simulink model "VAB_Linear_Discrete_Piffo"  (R2019b)
settings: Solver=VariableStepAuto  StartTime=0.0  StopTime=t_end  FixedStep=Ts  RelTol=1e-3
undefined symbols (not defined in the file): A_real, B_real, C_real, phi_p_setpoint, Ts, x_0
settings Model: EnablePacing=on  PacingRate=0.045000  Creator=miche  LastModifiedBy=miche

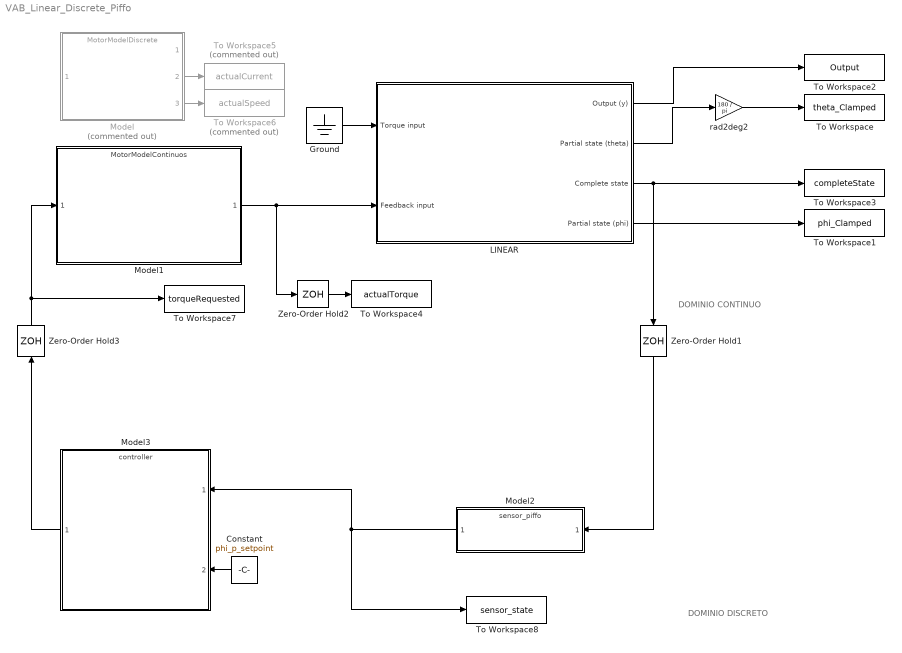
== system VAB_Linear_Discrete_Piffo ==
  note: DOMINIO CONTINUO
  note: DOMINIO DISCRETO
  Constant : Constant  Value=phi_p_setpoint
  Ground : Ground
  LINEAR : Subsystem
  Model : ModelReference  Commented=on  ModelNameDialog=MotorModelDiscrete.slx  SimulationMode=Normal  ModelReferenceVersion=1.14
  Model1 : ModelReference  ModelNameDialog=MotorModelContinuos.slx  SimulationMode=Normal  ModelReferenceVersion=1.24
  Model2 : ModelReference  ModelNameDialog=sensor_piffo.slx  SimulationMode=Normal  ModelReferenceVersion=1.14
  Model3 : ModelReference  ModelNameDialog=controller.slx  SimulationMode=Normal  ModelReferenceVersion=1.20
  To Workspace : ToWorkspace  VariableName=theta_Clamped  SampleTime=-1
  To Workspace1 : ToWorkspace  VariableName=phi_Clamped  SampleTime=-1
  To Workspace2 : ToWorkspace  VariableName=Output  SampleTime=-1
  To Workspace3 : ToWorkspace  VariableName=completeState  SampleTime=-1
  To Workspace4 : ToWorkspace  VariableName=actualTorque  SampleTime=-1
  To Workspace5 : ToWorkspace  Commented=on  VariableName=actualCurrent  SampleTime=-1
  To Workspace6 : ToWorkspace  Commented=on  VariableName=actualSpeed  SampleTime=-1
  To Workspace7 : ToWorkspace  VariableName=torqueRequested  SampleTime=-1
  To Workspace8 : ToWorkspace  VariableName=sensor_state  SampleTime=-1
  Zero-Order Hold1 : ZeroOrderHold  SampleTime=Ts
  Zero-Order Hold2 : ZeroOrderHold  SampleTime=Ts
  Zero-Order Hold3 : ZeroOrderHold  SampleTime=Ts
  rad2deg2 : Gain  Gain=180 / pi
  wires:
  LINEAR/2(Partial state (theta)) -> rad2deg2/1
  LINEAR/1(Output (y)) -> To Workspace2/1
  LINEAR/3("Complete state ") -> Zero-Order Hold1/1, To Workspace3/1
  LINEAR/4(Partial state (phi)) -> To Workspace1/1
  rad2deg2/1 -> To Workspace/1
  Model/2 -> To Workspace5/1
  Model/3 -> To Workspace6/1
  Model3/1 -> Zero-Order Hold3/1
  Model1/1 -> LINEAR/2(Feedback input), Zero-Order Hold2/1
  Zero-Order Hold2/1 -> To Workspace4/1
  Zero-Order Hold1/1 -> Model2/1
  Constant/1 -> Model3/2
  Zero-Order Hold3/1 -> To Workspace7/1, Model1/1
  Ground/1 -> LINEAR/1(Torque input)
  Model2/1 -> To Workspace8/1, Model3/1

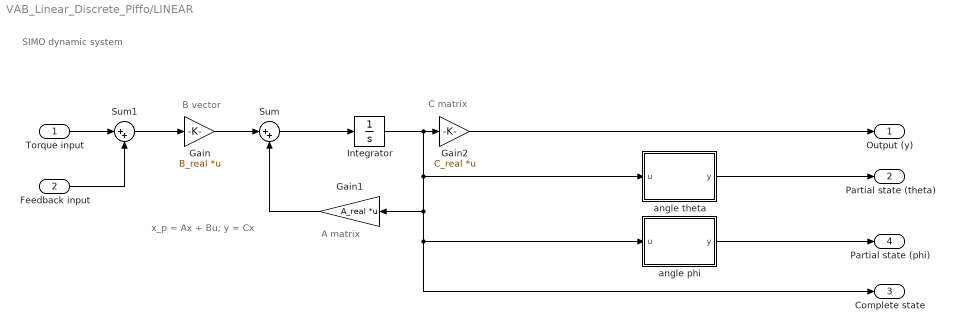
== system VAB_Linear_Discrete_Piffo/LINEAR ==
  note: C matrix
  note: SIMO dynamic system
  note: x_p = Ax + Bu;
      | y = Cx
  note: B vector
  note: A matrix
  Torque input : Inport
  Feedback input : Inport  Port=2
  Gain : Gain  Gain=B_real  Multiplication=Matrix(K*u) (u vector)
  Gain1 : Gain  Gain=A_real  Multiplication=Matrix(K*u) (u vector)
  Gain2 : Gain  Gain=C_real  Multiplication=Matrix(K*u) (u vector)
  Integrator : Integrator  InitialCondition=x_0
  Sum : Sum  Inputs=|++
  Sum1 : Sum  Inputs=|++
  angle phi : MATLAB Function  TreatAsAtomicUnit=on
  angle theta : MATLAB Function  TreatAsAtomicUnit=on
  Output (y) : Outport
  Partial state (theta) : Outport  Port=2
  "Complete state " : Outport  Port=3
  Partial state (phi) : Outport  Port=4
  wires:
  Gain2/1 -> Output (y)/1
  Gain1/1 -> Sum/2
  Gain/1 -> Sum/1
  Sum/1 -> Integrator/1
  Sum1/1 -> Gain/1
  Feedback input/1 -> Sum1/2
  Torque input/1 -> Sum1/1
  Integrator/1 -> Gain2/1, angle theta/1(u), angle phi/1(u), "Complete state "/1, Gain1/1
  angle phi/1(y) -> Partial state (phi)/1
  angle theta/1(y) -> Partial state (theta)/1

== matlab function VAB_Linear_Discrete_Piffo/LINEAR/angle phi ==
  data: u input; y output
function y = fcn(u)

% if u(1) ~= 0
%    u(1) = mod(u(1), 2 * pi); 
% end
% 
% y = rad2deg(u(1));
y = u(1);

== matlab function VAB_Linear_Discrete_Piffo/LINEAR/angle theta ==
  data: u input; y output
function y = fcn(u)

% if u(3) ~= 0
%    u(3) = mod(u(3), 2 * pi); 
% end
% 
% 
% y = rad2deg(u(3));
y = u(3);
